simulink model "System_Modell"  (R2018a)
settings: Solver=FixedStepAuto  StartTime=0.0  StopTime=inf  FixedStep=1/f  RelTol=1e-3
values from neighbouring files (symbols this model uses):
  f = 10000    [System_Init.m]
(part 8 of 8)

== matlab function System_Modell/Motor_3/Schnittstelle_0/Send_to_Host ==
  data: signal output boolean size=1; package output double; Recv_Buffer data_store_memory; Filter data_store_memory; lenR input; lenF input; signal_old input
% Name: Send_to_Host
% Funktionalitäten:
% 1. Erste Zeile der Nachricht von Recv_Buffer in Filter prüfen
% 2. nicht wiederholte Nachricht an Host senden
% 3. wiederholte Nachricht in Filter löschen
% 4. gesendete Nachricht in Filter kopieren
% 5. folgende Nachrichten eine Zeile nach oben verschoben


function [signal, package] = send_to_Host(lenR, lenF, signal_old)

global Recv_Buffer          % Package-List, which will be sent to the Host
global Filter               % Package-List, which has been sent to the Host

package = zeros(1,7);
check = 0;

if signal_old               % signal can only last for one periode
    signal = false;
    package = zeros(1,7);

else                        % signal inactiv --> now we can send new data to host.
    if (lenR >= 1)
        if lenF >= 1        % check in Filter
            for i=1:lenF        % check if the same message sent before
                if isequal(Recv_Buffer(1,:),Filter(i,:))
                    check = i;
                    break
                else
                    check = 0;
                end
            end
        end
        
        if check ~= 0       % same message in Filter found --> delete the message in Recv_Buffer and Filter
            signal = false;
            package = zeros(1,7);
            Filter(check:lenF-1,:) = Filter(check+1:lenF,:);
            Filter(lenF,:) = zeros(1,7);
            Recv_Buffer(1:lenR-1,:) = Recv_Buffer(2:lenR,:);
            Recv_Buffer(lenR,:) = zeros(1,7);
        else                % same message in Filter not found --> send to Host --> copy the message in Filter delete it in Recv_Buffer
            package = Recv_Buffer(1,:);
            signal = true;
            Filter(lenF+1,:) = Recv_Buffer(1,:);    % copy
            Recv_Buffer(1:lenR-1,:) = Recv_Buffer(2:lenR,:);    % delete
            Recv_Buffer(lenR,:) = zeros(1,7);
        end
    else
        signal = false;
        package = zeros(1,7);
    end
end


end

== stateflow chart System_Modell/Motor_3/Schnittstelle_0/Status ==
  state Init_0
    entry:	status=0;
    Handshake_1=false;
    Handshake_2=false;
    De_1 = 0;
    De_2 = 0;
    De_sum_1 = 0;
    De_sum_2 = 0;
    Filter(1,:) = zeros(1,7);
  state Error
    entry: status=-2;
  note: 未初始化全局变量
  state Init_1_Handshake
    entry: status=1;
  state Init_2_Delay_Time
    entry:	status=2;
  state Init_3_Sum_Delay_Time
    entry:	status=3;
  state Run
    entry: status=4;
  (default) -> Init_0
  Error -> Init_0 : [~Error_Signal]
  Init_0 -> Init_1_Handshake
  Init_1_Handshake -> Error [order 3] : [Error_Signal]
  Init_1_Handshake -> (junction 75) [order 1] : [recv_signal_1]
  (junction 75) -> Init_1_Handshake : [recv_data_1(1,3)==104]{Handshake_1 = true;}
  Init_1_Handshake -> (junction 77) [order 2] : [recv_signal_2]
  (junction 77) -> Init_1_Handshake : [recv_data_2(1,3)==104]{Handshake_2 = true;}
  Init_1_Handshake -> Init_2_Delay_Time [order 4] : [Handshake_1 && Handshake_2 && Address_1 > 0 && Address_2 > 0]
  Init_2_Delay_Time -> Error [order 2] : [Error_Signal]
  Init_2_Delay_Time -> Init_3_Sum_Delay_Time [order 1] : [De_1>0 && De_2>0]
  Init_3_Sum_Delay_Time -> Error [order 2] : [Error_Signal]
  Init_3_Sum_Delay_Time -> Run [order 1] : [De_sum_1 > De_1 && De_sum_2 > De_2]
  Run -> Error : [Error_Signal]
  data: status output double size=1; Error_Signal input boolean size=1; recv_signal_1 input boolean size=1; recv_data_1 input double; Handshake_1 data_store_memory size=1; Handshake_2 data_store_memory size=1; De_1 data_store_memory; De_2 data_store_memory; De_sum_1 data_store_memory; De_sum_2 data_store_memory; recv_signal_2 input boolean; recv_data_2 input double; Address_1 data_store_memory; Address_2 data_store_memory; Filter data_store_memory
